simulink model "beamformer_final"  (R2019b)
settings: Solver=VariableStepAuto  StartTime=0.0  StopTime=8  RelTol=1e-3
undefined symbols (not defined in the file or in its folder): mp
libraries: hdlsllib x9, simulink x1
settings Model: Creator=khristian  LastModifiedBy=jones
settings DataIOCC: ReturnWorkspaceOutputs=off
settings OptimizationCC: BlockReduction=off  ConditionallyExecuteInputs=off  DefaultParameterBehavior=Inlined
settings DebuggingCC: AlgebraicLoopMsg=error  ArithmeticOperatorsInVariantConditions=warning
settings HardwareCC: ProdBitPerPointer=32  ProdBitPerSizeT=32  ProdBitPerPtrDiffT=32  ProdLargestAtomicFloat=None  ProdIntDivRoundTo=Undefined  ProdEndianess=Unspecified  ProdWordSize=32  ProdHWDeviceType=ASIC/FPGA->ASIC/FPGA  TargetBitPerPointer=64  TargetBitPerSizeT=64  TargetBitPerPtrDiffT=64  TargetLongLongMode=on  TargetIntDivRoundTo=Zero  TargetEndianess=LittleEndian  TargetWordSize=64  TargetHWDeviceType=Custom Processor->MATLAB Host Computer  ProdEqTarget=off
settings SFSimCC: CustomCodeUndefinedFunction=UseInterfaceOnly

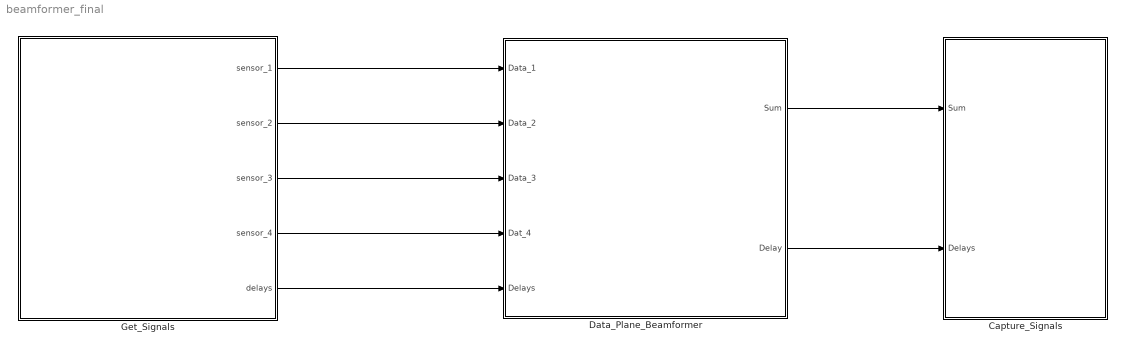
== system beamformer_final ==
  Capture_Signals : Subsystem
  Data_Plane_Beamformer : Subsystem
  Get_Signals : Subsystem
  wires:
  Get_Signals/1(sensor_1) -> Data_Plane_Beamformer/1(Data_1)
  Get_Signals/2(sensor_2) -> Data_Plane_Beamformer/2(Data_2)
  Get_Signals/4(sensor_4) -> Data_Plane_Beamformer/4(Dat_4)
  Get_Signals/5(delays) -> Data_Plane_Beamformer/5(Delays)
  Get_Signals/3(sensor_3) -> Data_Plane_Beamformer/3(Data_3)
  Data_Plane_Beamformer/1(Sum) -> Capture_Signals/1(Sum)
  Data_Plane_Beamformer/2(Delay) -> Capture_Signals/2(Delays)

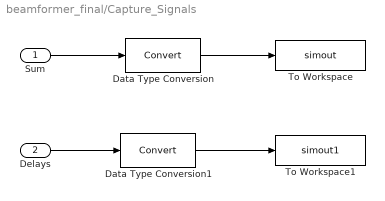
== system beamformer_final/Capture_Signals ==
  Sum : Inport
  Delays : Inport  Port=2
  Data Type Conversion : DataTypeConversion
  Data Type Conversion1 : DataTypeConversion
  To Workspace : ToWorkspace  VariableName=simout  SaveFormat=Timeseries  SampleTime=-1
  To Workspace1 : ToWorkspace  VariableName=simout1  SaveFormat=Timeseries  SampleTime=-1
  wires:
  Sum/1 -> Data Type Conversion/1
  Delays/1 -> Data Type Conversion1/1
  Data Type Conversion/1 -> To Workspace/1
  Data Type Conversion1/1 -> To Workspace1/1

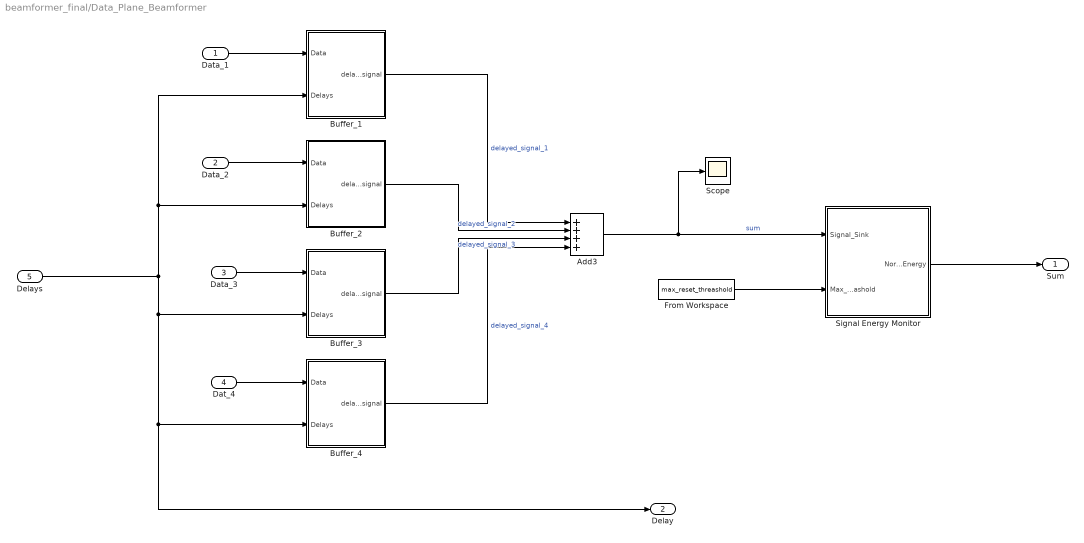
== system beamformer_final/Data_Plane_Beamformer ==
  Data_1 : Inport
  Data_2 : Inport  Port=2
  Data_3 : Inport  Port=3
  Dat_4 : Inport  Port=4
  Delays : Inport  Port=5
  Add3 : Sum  Inputs=++++
  Buffer_1 : Subsystem
  Buffer_2 : Subsystem
  Buffer_3 : Subsystem
  Buffer_4 : Subsystem
  From Workspace : FromWorkspace  VariableName=max_reset_threashold  SampleTime=0
  Scope : Scope
  Signal Energy Monitor : Subsystem
  Sum : Outport  VectorParamsAs1DForOutWhenUnconnected=off
  Delay : Outport  Port=2  VectorParamsAs1DForOutWhenUnconnected=off
  wires:
  Buffer_1/1(delayed_signal) -> Add3/1  "delayed_signal_1"
  Buffer_4/1(delayed_signal) -> Add3/4  "delayed_signal_4"
  Add3/1 -> Signal Energy Monitor/1("Signal_Sink "), Scope/1  "sum"
  Buffer_3/1(delayed_signal) -> Add3/3  "delayed_signal_3"
  Data_3/1 -> Buffer_3/1(Data)
  Dat_4/1 -> Buffer_4/1(Data)
  Buffer_2/1(delayed_signal) -> Add3/2  "delayed_signal_2"
  Data_2/1 -> Buffer_2/1(Data)
  Delays/1 -> Buffer_2/2(Delays), Buffer_1/2(Delays), Buffer_3/2(Delays), Buffer_4/2(Delays), Delay/1
  Data_1/1 -> Buffer_1/1(Data)
  Signal Energy Monitor/1(Normalized_Signal_Energy) -> Sum/1
  From Workspace/1 -> Signal Energy Monitor/2(Max_Reset_Threashold)

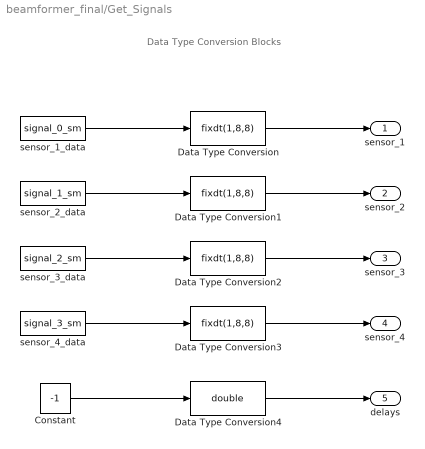
== system beamformer_final/Get_Signals ==
  note: Data Type Conversion Blocks
  Constant : Constant  Value=-1  SampleTime=-1
  Data Type Conversion{,1..3} (4 alike) : DataTypeConversion  OutDataTypeStr=fixdt(1,8,8)
  Data Type Conversion4 : DataTypeConversion  OutDataTypeStr=double
  sensor_1_data : FromWorkspace  VariableName=signal_0_sm  SampleTime=0
  sensor_2_data : FromWorkspace  VariableName=signal_1_sm  SampleTime=0
  sensor_3_data : FromWorkspace  VariableName=signal_2_sm  SampleTime=0
  "sensor_4_data " : FromWorkspace  VariableName=signal_3_sm  SampleTime=0
  sensor_1 : Outport
  sensor_2 : Outport  Port=2  VectorParamsAs1DForOutWhenUnconnected=off
  sensor_3 : Outport  Port=3  VectorParamsAs1DForOutWhenUnconnected=off
  sensor_4 : Outport  Port=4  VectorParamsAs1DForOutWhenUnconnected=off
  delays : Outport  Port=5  VectorParamsAs1DForOutWhenUnconnected=off
  wires:
  sensor_1_data/1 -> Data Type Conversion/1
  sensor_2_data/1 -> Data Type Conversion1/1
  sensor_3_data/1 -> Data Type Conversion2/1
  "sensor_4_data "/1 -> Data Type Conversion3/1
  Data Type Conversion/1 -> sensor_1/1
  Data Type Conversion1/1 -> sensor_2/1
  Data Type Conversion2/1 -> sensor_3/1
  Data Type Conversion3/1 -> sensor_4/1
  Data Type Conversion4/1 -> delays/1
  Constant/1 -> Data Type Conversion4/1

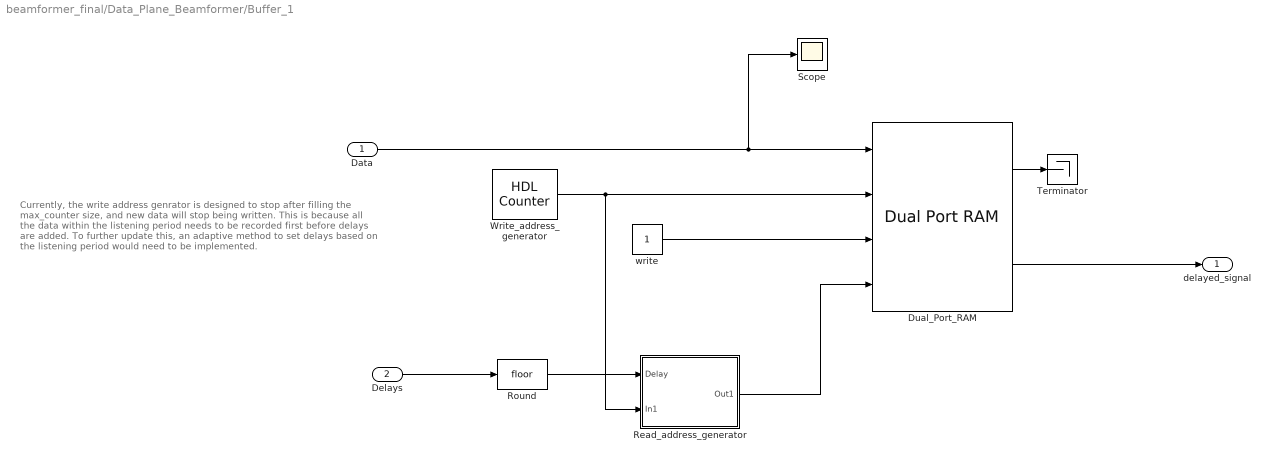
== system beamformer_final/Data_Plane_Beamformer/Buffer_1 ==
  note: Currently, the write  address genrator is designed to
      | stop after filling the max_counter
      | size, and new data will stop being written.
      | This is because all the data within the listening period
      | needs to be recorded first before delays are added.
      | To further update this, an adaptive method to set delays
      | based on the listening period
      | would need to be implemented.
  Data : Inport
  Delays : Inport  Port=2
  Dual_Port_RAM : hdlsllib/HDL RAMs/Dual Port RAM  ram_size=13
      settings: SourceProductName=Simulink  SourceProductBaseCode=SL
  Read_address_generator : Subsystem
  Round : Rounding
  Scope : Scope
  Terminator : Terminator
  Write_address_generator : hdlsllib/Sources/HDL Counter  CountType=Count limited  CountInit=0  CountStep=1  CountMax=8191  CountFromType=Initial value  CountFrom=0  CountResetPort=off  CountLoadPort=off  CountEnbPort=off  CountDirPort=off  CountDataType=Unsigned  CountWordLen=13  CountFracLen=0  CountSampTime=1/200
      settings: SourceProductName=Simulink
  write : Constant  OutDataTypeStr=boolean  SampleTime=-1
  delayed_signal : Outport  VectorParamsAs1DForOutWhenUnconnected=off
  wires:
  Write_address_generator/1 -> Read_address_generator/2(In1), Dual_Port_RAM/2
  Data/1 -> Scope/1, Dual_Port_RAM/1
  Read_address_generator/1(Out1) -> Dual_Port_RAM/4
  Dual_Port_RAM/2 -> delayed_signal/1
  Dual_Port_RAM/1 -> Terminator/1
  Delays/1 -> Round/1
  write/1 -> Dual_Port_RAM/3
  Round/1 -> Read_address_generator/1(Delay)

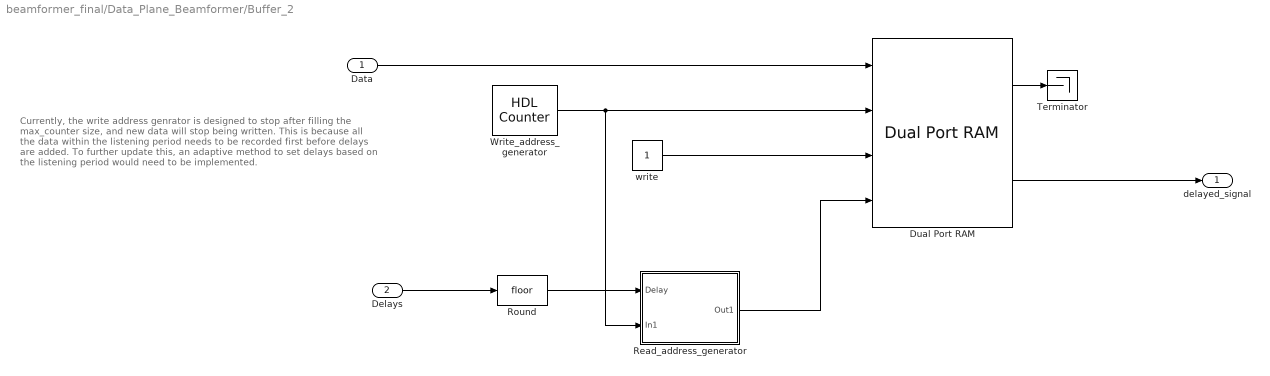
== system beamformer_final/Data_Plane_Beamformer/Buffer_2 ==
  note: Currently, the write  address genrator is designed to
      | stop after filling the max_counter
      | size, and new data will stop being written.
      | This is because all the data within the listening period
      | needs to be recorded first before delays are added.
      | To further update this, an adaptive method to set delays
      | based on the listening period
      | would need to be implemented.
  Data : Inport
  Delays : Inport  Port=2
  Dual Port RAM : hdlsllib/HDL RAMs/Dual Port RAM  ram_size=13
      settings: SourceProductName=Simulink  SourceProductBaseCode=SL
  Read_address_generator : Subsystem
  Round : Rounding
  Terminator : Terminator
  Write_address_generator : hdlsllib/Sources/HDL Counter  CountType=Count limited  CountInit=0  CountStep=1  CountMax=8191  CountFromType=Initial value  CountFrom=0  CountResetPort=off  CountLoadPort=off  CountEnbPort=off  CountDirPort=off  CountDataType=Unsigned  CountWordLen=13  CountFracLen=0  CountSampTime=1/200
      settings: SourceProductName=Simulink
  write : Constant  OutDataTypeStr=boolean  SampleTime=-1
  delayed_signal : Outport  VectorParamsAs1DForOutWhenUnconnected=off
  wires:
  Write_address_generator/1 -> Read_address_generator/2(In1), Dual Port RAM/2
  Data/1 -> Dual Port RAM/1
  Read_address_generator/1(Out1) -> Dual Port RAM/4
  Dual Port RAM/2 -> delayed_signal/1
  Dual Port RAM/1 -> Terminator/1
  Delays/1 -> Round/1
  write/1 -> Dual Port RAM/3
  Round/1 -> Read_address_generator/1(Delay)

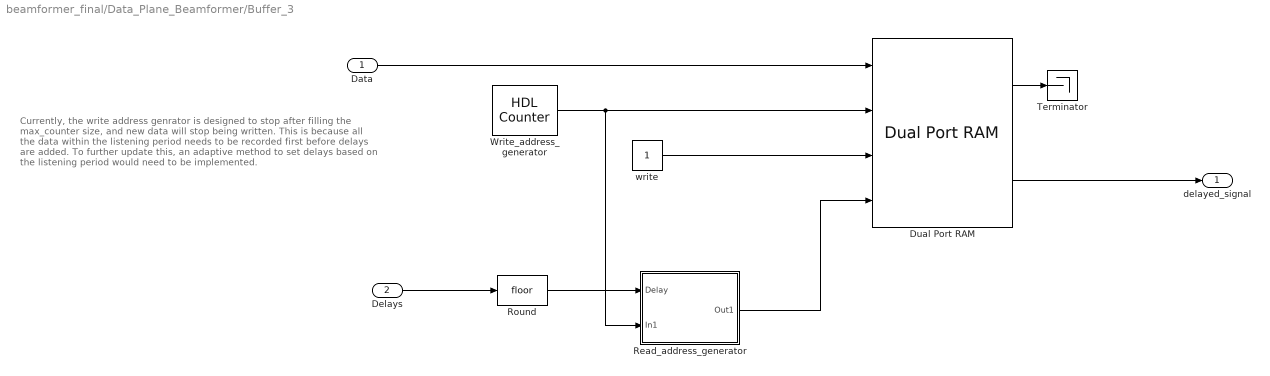
== system beamformer_final/Data_Plane_Beamformer/Buffer_3 ==
  note: Currently, the write  address genrator is designed to
      | stop after filling the max_counter
      | size, and new data will stop being written.
      | This is because all the data within the listening period
      | needs to be recorded first before delays are added.
      | To further update this, an adaptive method to set delays
      | based on the listening period
      | would need to be implemented.
  Data : Inport
  Delays : Inport  Port=2
  Dual Port RAM : hdlsllib/HDL RAMs/Dual Port RAM  ram_size=13
      settings: SourceProductName=Simulink  SourceProductBaseCode=SL
  Read_address_generator : Subsystem
  Round : Rounding
  Terminator : Terminator
  Write_address_generator : hdlsllib/Sources/HDL Counter  CountType=Count limited  CountInit=0  CountStep=1  CountMax=8191  CountFromType=Initial value  CountFrom=0  CountResetPort=off  CountLoadPort=off  CountEnbPort=off  CountDirPort=off  CountDataType=Unsigned  CountWordLen=13  CountFracLen=0  CountSampTime=1/200
      settings: SourceProductName=Simulink
  write : Constant  OutDataTypeStr=boolean  SampleTime=-1
  delayed_signal : Outport  VectorParamsAs1DForOutWhenUnconnected=off
  wires:
  Write_address_generator/1 -> Read_address_generator/2(In1), Dual Port RAM/2
  Data/1 -> Dual Port RAM/1
  Read_address_generator/1(Out1) -> Dual Port RAM/4
  Dual Port RAM/2 -> delayed_signal/1
  Dual Port RAM/1 -> Terminator/1
  Delays/1 -> Round/1
  write/1 -> Dual Port RAM/3
  Round/1 -> Read_address_generator/1(Delay)

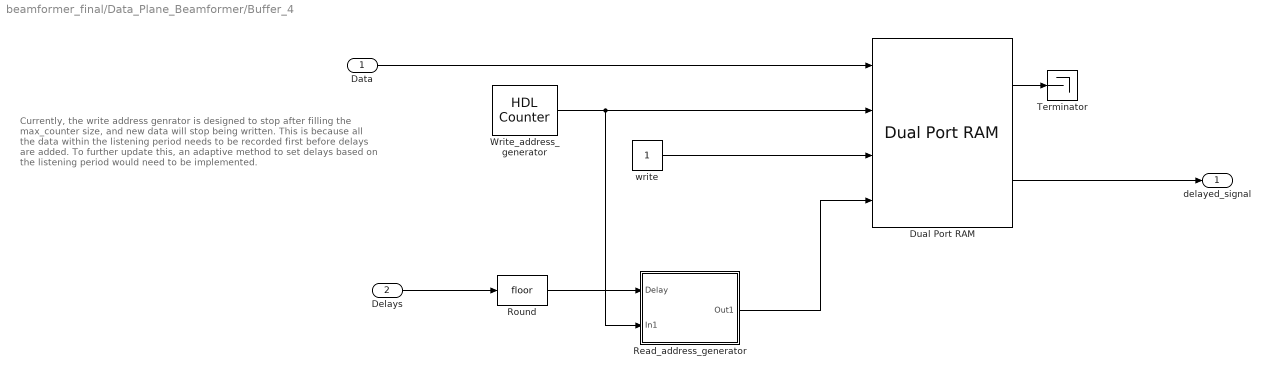
== system beamformer_final/Data_Plane_Beamformer/Buffer_4 ==
  note: Currently, the write  address genrator is designed to
      | stop after filling the max_counter
      | size, and new data will stop being written.
      | This is because all the data within the listening period
      | needs to be recorded first before delays are added.
      | To further update this, an adaptive method to set delays
      | based on the listening period
      | would need to be implemented.
  Data : Inport
  Delays : Inport  Port=2
  Dual Port RAM : hdlsllib/HDL RAMs/Dual Port RAM  ram_size=13
      settings: SourceProductName=Simulink  SourceProductBaseCode=SL
  Read_address_generator : Subsystem
  Round : Rounding
  Terminator : Terminator
  Write_address_generator : hdlsllib/Sources/HDL Counter  CountType=Count limited  CountInit=0  CountStep=1  CountMax=8191  CountFromType=Initial value  CountFrom=0  CountResetPort=off  CountLoadPort=off  CountEnbPort=off  CountDirPort=off  CountDataType=Unsigned  CountWordLen=13  CountFracLen=0  CountSampTime=1/200
      settings: SourceProductName=Simulink
  write : Constant  OutDataTypeStr=boolean  SampleTime=-1
  delayed_signal : Outport  VectorParamsAs1DForOutWhenUnconnected=off
  wires:
  Write_address_generator/1 -> Read_address_generator/2(In1), Dual Port RAM/2
  Data/1 -> Dual Port RAM/1
  Read_address_generator/1(Out1) -> Dual Port RAM/4
  Dual Port RAM/2 -> delayed_signal/1
  Dual Port RAM/1 -> Terminator/1
  Delays/1 -> Round/1
  write/1 -> Dual Port RAM/3
  Round/1 -> Read_address_generator/1(Delay)

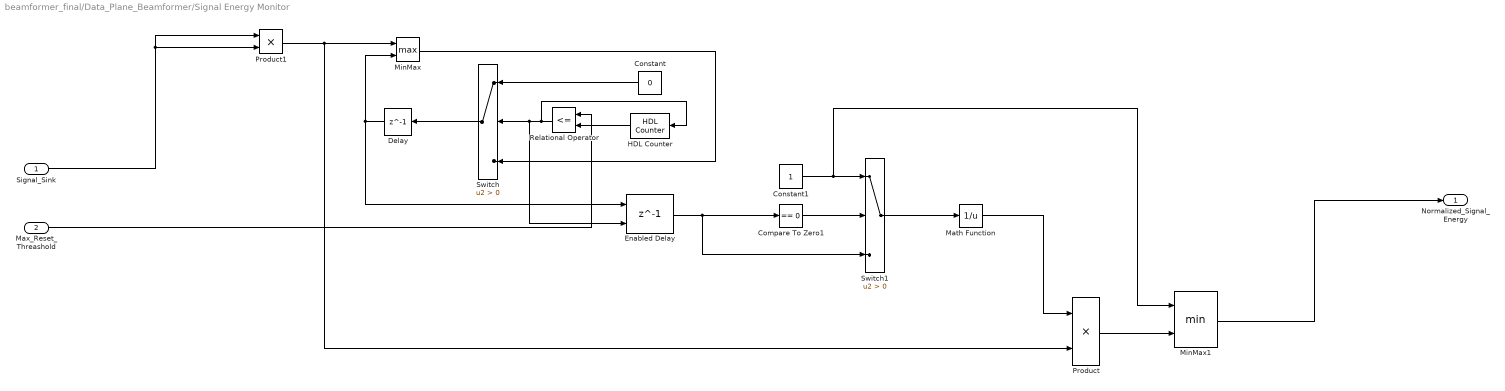
== system beamformer_final/Data_Plane_Beamformer/Signal Energy Monitor ==
  "Signal_Sink " : Inport
  Max_Reset_Threashold : Inport  Port=2
  Compare To Zero1 : simulink/Logic and Bit Operations/Compare To Zero  relop===  OutDataTypeStr=boolean
  Constant : Constant  Value=0  OutDataTypeStr=fixdt(1,mp.W_bits,mp.F_bits)  SampleTime=mp.Ts_system
  Constant1 : Constant  OutDataTypeStr=fixdt(1,mp.W_bits, mp.F_bits)  SampleTime=mp.Ts_system
  Delay : Delay  DelayLength=1
  Enabled Delay : Delay  DelayLength=1  ShowEnablePort=on
      settings: InputPortMap=u0,e6
  HDL Counter : hdlsllib/Sources/HDL Counter  CountType=Free running  CountInit=0  CountStep=1  CountMax=25  CountFromType=Initial value  CountFrom=0  CountResetPort=on  CountLoadPort=off  CountEnbPort=off  CountDirPort=off  CountDataType=Unsigned  CountWordLen=mp.max_reset_Nbits  CountFracLen=1  CountSampTime=1
      settings: SourceProductName=Simulink
  Math Function : Math  Operator=reciprocal  RndMeth=Zero  SaturateOnIntegerOverflow=on
  MinMax : MinMax  Function=max  Inputs=2
  MinMax1 : MinMax  Inputs=2
  Product : Product
  Product1 : Product  OutDataTypeStr=fixdt(1, mp.W_bits, mp.F_bits)
  Relational Operator : RelationalOperator  Operator=<=  OutDataTypeStr=boolean  RndMeth=Nearest
  Switch : Switch  Criteria=u2 > Threshold
  Switch1 : Switch  Criteria=u2 > Threshold
  Normalized_Signal_Energy : Outport  VectorParamsAs1DForOutWhenUnconnected=off
  wires:
  MinMax1/1 -> Normalized_Signal_Energy/1
  Max_Reset_Threashold/1 -> Relational Operator/1
  "Signal_Sink "/1 -> Product1/2, Product1/1
  Product/1 -> MinMax1/2
  Math Function/1 -> Product/1
  Constant1/1 -> MinMax1/1, Switch1/1
  Constant/1 -> Switch/1
  Delay/1 -> Enabled Delay/1, MinMax/2
  Product1/1 -> Product/2, MinMax/1
  HDL Counter/1 -> Relational Operator/2
  Switch1/1 -> Math Function/1
  MinMax/1 -> Switch/3
  Relational Operator/1 -> HDL Counter/1, Enabled Delay/2, Switch/2
  Enabled Delay/1 -> Switch1/3, Compare To Zero1/1
  Switch/1 -> Delay/1
  Compare To Zero1/1 -> Switch1/2

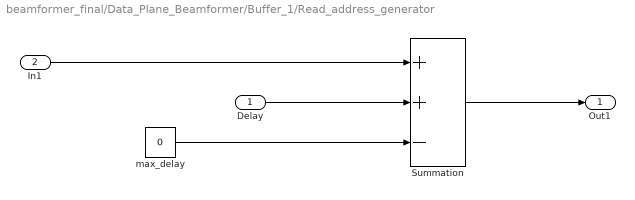
== system beamformer_final/Data_Plane_Beamformer/Buffer_1/Read_address_generator ==
  Delay : Inport
  In1 : Inport  Port=2
  Summation : Sum  Inputs=++-  OutDataTypeStr=fixdt(0,13,0)
  max_delay : Constant  Value=0  SampleTime=-1
  Out1 : Outport
  wires:
  In1/1 -> Summation/1
  Delay/1 -> Summation/2
  Summation/1 -> Out1/1
  max_delay/1 -> Summation/3

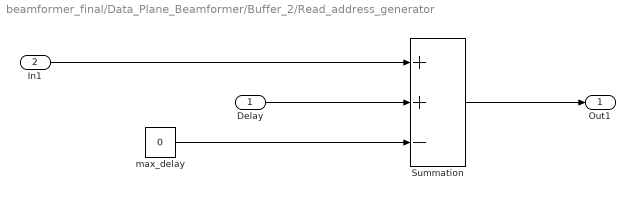
== system beamformer_final/Data_Plane_Beamformer/Buffer_2/Read_address_generator ==
  Delay : Inport
  In1 : Inport  Port=2
  Summation : Sum  Inputs=++-  OutDataTypeStr=fixdt(0,13,0)
  max_delay : Constant  Value=0  SampleTime=-1
  Out1 : Outport
  wires:
  In1/1 -> Summation/1
  Delay/1 -> Summation/2
  Summation/1 -> Out1/1
  max_delay/1 -> Summation/3

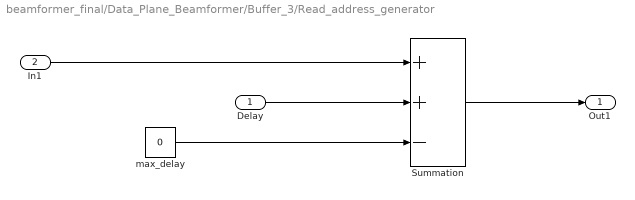
== system beamformer_final/Data_Plane_Beamformer/Buffer_3/Read_address_generator ==
  Delay : Inport
  In1 : Inport  Port=2
  Summation : Sum  Inputs=++-  OutDataTypeStr=fixdt(0,13,0)
  max_delay : Constant  Value=0  SampleTime=-1
  Out1 : Outport
  wires:
  In1/1 -> Summation/1
  Delay/1 -> Summation/2
  Summation/1 -> Out1/1
  max_delay/1 -> Summation/3

== system beamformer_final/Data_Plane_Beamformer/Buffer_4/Read_address_generator ==
  Delay : Inport
  In1 : Inport  Port=2
  Summation : Sum  Inputs=++-  OutDataTypeStr=fixdt(0,13,0)
  max_delay : Constant  Value=0  SampleTime=-1
  Out1 : Outport
  wires:
  In1/1 -> Summation/1
  Delay/1 -> Summation/2
  Summation/1 -> Out1/1
  max_delay/1 -> Summation/3
